simulink model "optimized_pwm"  (R2017a)
settings: Solver=VariableStepAuto  StartTime=0.0  StopTime=0.5  MaxStep=1e-4  RelTol=1e-3
libraries: powerlib x10, simulink x2
settings Model: Creator=lenovo 520  LastModifiedBy=lenovo 520

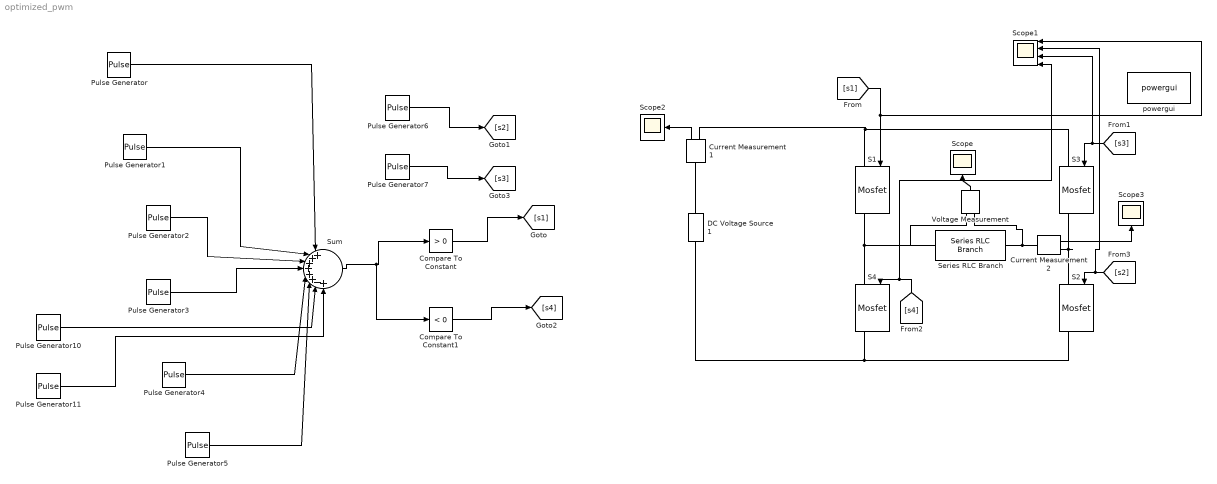
== system optimized_pwm ==
  Compare To Constant : simulink/Logic and Bit Operations/Compare To Constant  relop=>  const=0  OutDataTypeStr=boolean
  Compare To Constant1 : simulink/Logic and Bit Operations/Compare To Constant  relop=<  const=0  OutDataTypeStr=boolean
  Current Measurement1 : powerlib/Measurements/Current Measurement  PhasorSimulation=off  OutputType=Complex  PSBequivalent=0
  Current Measurement2 : powerlib/Measurements/Current Measurement  PhasorSimulation=off  OutputType=Complex  PSBequivalent=0
  DC Voltage Source 1 : powerlib/Electrical Sources/DC Voltage Source  Amplitude=200  Measurements=None
  Pulse Generator : DiscretePulseGenerator  PulseType=Time based  Period=0.02  PulseWidth=5.7756  PhaseDelay=1.46889e-3
  Pulse Generator1 : DiscretePulseGenerator  PulseType=Time based  Period=0.02  PulseWidth=19.2633  PhaseDelay=3.0731667e-3
  Pulse Generator10 : DiscretePulseGenerator  PulseType=Time based  Amplitude=0.1  Period=0.02  PulseWidth=50
  Pulse Generator11 : DiscretePulseGenerator  PulseType=Time based  Amplitude=0.1  Period=0.02  PulseWidth=50  PhaseDelay=0.01
  Pulse Generator2 : DiscretePulseGenerator  PulseType=Time based  Period=0.02  PulseWidth=5.77556  PhaseDelay=7.376e-3
  Pulse Generator3 : DiscretePulseGenerator  PulseType=Time based  Amplitude=-1  Period=0.02  PulseWidth=5.7756  PhaseDelay=1.46889e-3+0.01
  Pulse Generator4 : DiscretePulseGenerator  PulseType=Time based  Amplitude=-1  Period=0.02  PulseWidth=19.2633  PhaseDelay=3.0731667e-3+0.01
  Pulse Generator5 : DiscretePulseGenerator  PulseType=Time based  Amplitude=-1  Period=0.02  PulseWidth=5.77556  PhaseDelay=7.376e-3+0.01
  Pulse Generator6 : DiscretePulseGenerator  PulseType=Time based  Period=0.02  PulseWidth=50
  Pulse Generator7 : DiscretePulseGenerator  PulseType=Time based  Period=0.02  PulseWidth=50  PhaseDelay=0.01
  S{1..4} (4 alike) : powerlib/Power Electronics/Mosfet  Ron=0  Lon=0  Rd=0  Vfd=0  IC=0  Rs=1e5  Cs=inf  Measurements=on
  Scope : Scope
  Scope1 : Scope  NumInputPorts=4
  Scope2 : Scope
  Scope3 : Scope
  "Series RLC Branch " : powerlib/Elements/Series RLC Branch  LConnTagsString=__new0  RConnTagsString=__new0  BranchType=RLC  Resistance=1  Inductance=5e-3  SetiL0=off  InitialCurrent=0  Capacitance=0  Setx0=off  InitialVoltage=0  Measurements=None
  Sum : Sum  Inputs=|++++++-+
  Voltage Measurement : powerlib/Measurements/Voltage Measurement  PhasorSimulation=off  OutputType=Complex  PSBequivalent=0
  powergui : powerlib/powergui  Priority=1  SimulationMode=Continuous  SampleTime=50e-6  frequency=60  Iterations=50  frequencyindice=0  Pbase=100e6  ErrMax=1e-4  UnitsV=kV  UnitsW=MW  buscounter=0  FunctionMessages=off  echomessages=off  EnableUseOfTLC=off  CurrentSourceSwitches=off  DisableSnubberDevices=off  DisableRonSwitches=off  DisableVfSwitches=off  DisplayEquations=off  SolverType=Tustin/Backward Euler (TBE)  Interpol=off  ExternalGateDelay=off  methode=off  Ts=100  x0status=blocks  SPID=on  SwTol=0  HookPort=off  RestoreLinks=warning  ResistiveCurrentMeasurement=off  Frange=[0:2:500]  Ylog=off  Xlog=on  ShowGrid=off  save=off  variable=ZData  structure=curent  ZoomFFT=off  StartTime=0.08  cycles=10  DisplayStyle=1  fundamental=50  FreqAxis=off  MaxFrequency=500  frequencyindicesteady=1  RmsSteady=1  display=off
  wires:
  Current Measurement1/1 -> Scope2/1
  Pulse Generator/1 -> Sum/1
  Pulse Generator1/1 -> Sum/2
  Pulse Generator2/1 -> Sum/3
  Pulse Generator3/1 -> Sum/4
  Pulse Generator4/1 -> Sum/5
  Pulse Generator5/1 -> Sum/6
  Sum/1 -> Compare To Constant1/1, Compare To Constant/1
  Compare To Constant/1 -> [s1]
  Compare To Constant1/1 -> [s4]
  [s1] -> Scope1/1, S1/1
  [s3] -> Scope1/3, S3/1
  [s2] -> Scope1/2, S2/1
  [s4] -> Scope1/4, S4/1
  Voltage Measurement/1 -> Scope/1
  Pulse Generator6/1 -> [s2]
  Pulse Generator11/1 -> Sum/8
  Pulse Generator10/1 -> Sum/7
  Pulse Generator7/1 -> [s3]
  Current Measurement2/1 -> Scope3/1
  connections:
  S1/RConn1 -- Voltage Measurement/LConn1 -- "Series RLC Branch "/LConn1 -- S4/LConn1
  Voltage Measurement/LConn2 -- Current Measurement2/LConn1 -- "Series RLC Branch "/RConn1
  S3/LConn1 -- Current Measurement1/RConn1 -- S1/LConn1
  S2/RConn1 -- DC Voltage Source 1/LConn1 -- S4/RConn1
  Current Measurement1/LConn1 -- DC Voltage Source 1/RConn1
  S3/RConn1 -- S2/LConn1 -- Current Measurement2/RConn1
